simulink model "myrobot"  (R2019b)
settings: Solver=FixedStepAuto  StartTime=0.0  StopTime=2  FixedStep=0.001  MaxStep=0.005  RelTol=1e-3
values from neighbouring files (symbols this model uses):
  g = [0 0 -9.81]    [FK.m]    (also in FK_3DOF.m = [0 0 9.81])
  X = [joint1_pos(1) joint2_pos(1) joint3_pos(1) ee_pos(1)]    [plot_result.m]
  Y = [joint1_pos(2) joint2_pos(2) joint3_pos(2) ee_pos(2)]    [plot_result.m]
  Z = [joint1_pos(3) joint2_pos(3) joint3_pos(3) ee_pos(3)]    [plot_result.m]
libraries: sm_lib x17, nesl_utility x13, robotmaniplib x4, simulink x2
(part 2 of 7)

== matlab function myrobot/DYNAMICS SOLVER/MATLAB Function ==
  data: q input; q_dot input; M output; C output; G output
function [M,C,G] = calculate_dynamics(q,q_dot)

M_func = @(theta1,theta2,theta3)reshape([(sin(theta1).*(-2.272809781200003e-2)+cos(theta1).*sin(theta2).*2.2140098+cos(theta1).*cos(theta2).*sin(theta3).*6.228833385e-1+cos(theta1).*cos(theta3).*sin(theta2).*6.228833385e-1).*(sin(theta1).*(-4.414200000000005e-3)+cos(theta1).*sin(theta2).*(4.3e+1./1.0e+2)+cos(theta1).*cos(theta2).*sin(theta3).*1.20975e-1+cos(theta1).*cos(theta3).*sin(theta2).*1.20975e-1)+sin(theta2).*(cos(theta2).*1.41285e-7+sin(theta2).*2.5374e-1)+cos(theta1).^2.*1.922862803445e-4+sin(theta1).^2.*1.922862803445e-4+(cos(theta2).*cos(theta3)-sin(theta2).*sin(theta3)).*(cos(theta2).*cos(theta3).*1.0425e-2+cos(theta2).*sin(theta3).*2.67415e-8+cos(theta3).*sin(theta2).*2.67415e-8-sin(theta2).*sin(theta3).*1.0425e-2)+(cos(theta1).*2.272809781200003e-2+sin(theta1).*sin(theta2).*2.2140098+cos(theta2).*sin(theta1).*sin(theta3).*6.228833385e-1+cos(theta3).*sin(theta1).*sin(theta2).*6.228833385e-1).*(cos(theta1).*4.414200000000005e-3+sin(theta1).*sin(theta2).*(4.3e+1./1.0e+2)+cos(theta2).*sin(theta1).*sin(theta3).*1.20975e-1+cos(theta3).*sin(theta1).*sin(theta2).*1.20975e-1)+(sin(theta1).*1.4000105183-cos(theta1).*sin(theta2).*1.738546786).*(sin(theta1).*1.719281e-1-cos(theta1).*sin(theta2).*2.13502e-1)+(cos(theta1).*1.4000105183+sin(theta1).*sin(theta2).*1.738546786).*(cos(theta1).*1.719281e-1+sin(theta1).*sin(theta2).*2.13502e-1)+(cos(theta2).*sin(theta3)+cos(theta3).*sin(theta2)).*(cos(theta2).*cos(theta3).*2.67415e-8+cos(theta2).*sin(theta3).*7.5434e-2+cos(theta3).*sin(theta2).*7.5434e-2-sin(theta2).*sin(theta3).*2.67415e-8)+cos(theta2).*(cos(theta2).*2.12824e-2+sin(theta2).*1.41285e-7)+6.04953e-3,-sin(theta1).*((cos(theta2).*cos(theta3)-sin(theta2).*sin(theta3)).*(sin(theta1).*(-2.74946e-3)+cos(theta1).*sin(theta2).*sin(theta3).*2.67415e-8-cos(theta1).*cos(theta2).*cos(theta3).*2.67415e-8+cos(theta1).*cos(theta2).*sin(theta3).*1.0425e-2+cos(theta1).*cos(theta3).*sin(theta2).*1.0425e-2)+(cos(theta2).*sin(theta3)+cos(theta3).*sin(theta2)).*(sin(theta1).*(-2.13561e-9)+cos(theta1).*sin(theta2).*sin(theta3).*7.5434e-2-cos(theta1).*cos(theta2).*cos(theta3).*7.5434e-2+cos(theta1).*cos(theta2).*sin(theta3).*2.67415e-8+cos(theta1).*cos(theta3).*sin(theta2).*2.67415e-8))+cos(theta1).*((cos(theta2).*cos(theta3)-sin(theta2).*sin(theta3)).*(cos(theta1).*2.74946e-3+cos(theta2).*sin(theta1).*sin(theta3).*1.0425e-2+cos(theta3).*sin(theta1).*sin(theta2).*1.0425e-2+sin(theta1).*sin(theta2).*sin(theta3).*2.67415e-8-cos(theta2).*cos(theta3).*sin(theta1).*2.67415e-8)+(cos(theta2).*sin(theta3)+cos(theta3).*sin(theta2)).*(cos(theta1).*2.13561e-9+cos(theta2).*sin(theta1).*sin(theta3).*2.67415e-8+cos(theta3).*sin(theta1).*sin(theta2).*2.67415e-8+sin(theta1).*sin(theta2).*sin(theta3).*7.5434e-2-cos(theta2).*cos(theta3).*sin(theta1).*7.5434e-2))+sin(theta1).*(cos(theta2).*(sin(theta1).*4.99483e-3+cos(theta1).*cos(theta2).*1.41285e-7-cos(theta1).*sin(theta2).*2.12824e-2)-sin(theta2).*(sin(theta1).*7.13886e-8-cos(theta1).*cos(theta2).*2.5374e-1+cos(theta1).*sin(theta2).*1.41285e-7))+cos(theta1).*(cos(theta2).*(cos(theta1).*4.99483e-3-cos(theta2).*sin(theta1).*1.41285e-7+sin(theta1).*sin(theta2).*2.12824e-2)-sin(theta2).*(cos(theta1).*7.13886e-8+cos(theta2).*sin(theta1).*2.5374e-1-sin(theta1).*sin(theta2).*1.41285e-7))-(cos(theta1).*cos(theta2).*2.2140098-cos(theta1).*sin(theta2).*sin(theta3).*6.228833385e-1+cos(theta1).*cos(theta2).*cos(theta3).*6.228833385e-1).*(cos(theta1).*4.414200000000005e-3+sin(theta1).*sin(theta2).*(4.3e+1./1.0e+2)+cos(theta2).*sin(theta1).*sin(theta3).*1.20975e-1+cos(theta3).*sin(theta1).*sin(theta2).*1.20975e-1)+(cos(theta2).*sin(theta1).*2.2140098-sin(theta1).*sin(theta2).*sin(theta3).*6.228833385e-1+cos(theta2).*cos(theta3).*sin(theta1).*6.228833385e-1).*(sin(theta1).*(-4.414200000000005e-3)+cos(theta1).*sin(theta2).*(4.3e+1./1.0e+2)+cos(theta1).*cos(theta2).*sin(theta3).*1.20975e-1+cos(theta1).*cos(theta3).*sin(theta2).*1.20975e-1)-cos(theta1).*cos(theta2).*(cos(theta1).*1.719281e-1+sin(theta1).*sin(theta2).*2.13502e-1).*1.738546786-cos(theta2).*sin(theta1).*(sin(theta1).*1.719281e-1-cos(theta1).*sin(theta2).*2.13502e-1).*1.738546786,(cos(theta1).*sin(theta2).*sin(theta3).*6.228833385e-1-cos(theta1).*cos(theta2).*cos(theta3).*6.228833385e-1).*(cos(theta1).*4.414200000000005e-3+sin(theta1).*sin(theta2).*(4.3e+1./1.0e+2)+cos(theta2).*sin(theta1).*sin(theta3).*1.20975e-1+cos(theta3).*sin(theta1).*sin(theta2).*1.20975e-1)-(sin(theta1).*sin(theta2).*sin(theta3).*6.228833385e-1-cos(theta2).*cos(theta3).*sin(theta1).*6.228833385e-1).*(sin(theta1).*(-4.414200000000005e-3)+cos(theta1).*sin(theta2).*(4.3e+1./1.0e+2)+cos(theta1).*cos(theta2).*sin(theta3).*1.20975e-1+cos(theta1).*cos(theta3).*sin(theta2).*1.20975e-1)-sin(theta1).*((cos(theta2).*cos(theta3)-sin(theta2).*sin(theta3)).*(sin(theta1).*(-2.74946e-3)+cos(theta1).*sin(theta2).*sin(theta3).*2.67415e-8-cos(theta1).*cos(theta2).*cos(theta3).*2.67415e-8+cos(theta1).*cos(theta2).*sin(theta3).*1.0425e-2+cos(theta1).*cos(theta3).*sin(theta2).*1.0425e-2)+(cos(theta2).*sin(theta3)+cos(theta3).*sin(theta2)).*(sin(theta1).*(-2.13561e-9)+cos(theta1).*sin(theta2).*sin(theta3).*7.5434e-2-cos(theta1).*cos(theta2).*cos(theta3).*7.5434e-2+cos(theta1).*cos(theta2).*sin(theta3).*2.67415e-8+cos(theta1).*cos(theta3).*sin(theta2).*2.67415e-8))+cos(theta1).*((cos(theta2).*cos(theta3)-sin(theta2).*sin(theta3)).*(cos(theta1).*2.74946e-3+cos(theta2).*sin(theta1).*sin(theta3).*1.0425e-2+cos(theta3).*sin(theta1).*sin(theta2).*1.0425e-2+sin(theta1).*sin(theta2).*sin(theta3).*2.67415e-8-cos(theta2).*cos(theta3).*sin(theta1).*2.67415e-8)+(cos(theta2).*sin(theta3)+cos(theta3).*sin(theta2)).*(cos(theta1).*2.13561e-9+cos(theta2).*sin(theta1).*sin(theta3).*2.67415e-8+cos(theta3).*sin(theta1).*sin(theta2).*2.67415e-8+sin(theta1).*sin(theta2).*sin(theta3).*7.5434e-2-cos(theta2).*cos(theta3).*sin(theta1).*7.5434e-2)),cos(theta1).*(cos(theta1).*(cos(theta2).*cos(theta3).*2.74946e-3+cos(theta2).*sin(theta3).*2.13561e-9+cos(theta3).*sin(theta2).*2.13561e-9-sin(theta2).*sin(theta3).*2.74946e-3)+(cos(theta2).*sin(theta1).*sin(theta3)+cos(theta3).*sin(theta1).*sin(theta2)).*(cos(theta2).*cos(theta3).*1.0425e-2+cos(theta2).*sin(theta3).*2.67415e-8+cos(theta3).*sin(theta2).*2.67415e-8-sin(theta2).*sin(theta3).*1.0425e-2)+(sin(theta1).*sin(theta2).*sin(theta3)-cos(theta2).*cos(theta3).*sin(theta1)).*(cos(theta2).*cos(theta3).*2.67415e-8+cos(theta2).*sin(theta3).*7.5434e-2+cos(theta3).*sin(theta2).*7.5434e-2-sin(theta2).*sin(theta3).*2.67415e-8))-(cos(theta1).*cos(theta2).*(4.3e+1./1.0e+2)-cos(theta1).*sin(theta2).*sin(theta3).*1.20975e-1+cos(theta1).*cos(theta2).*cos(theta3).*1.20975e-1).*(cos(theta1).*2.272809781200003e-2+sin(theta1).*sin(theta2).*2.2140098+cos(theta2).*sin(theta1).*sin(theta3).*6.228833385e-1+cos(theta3).*sin(theta1).*sin(theta2).*6.228833385e-1)+(cos(theta2).*sin(theta1).*(4.3e+1./1.0e+2)-sin(theta1).*sin(theta2).*sin(theta3).*1.20975e-1+cos(theta2).*cos(theta3).*sin(theta1).*1.20975e-1).*(sin(theta1).*(-2.272809781200003e-2)+cos(theta1).*sin(theta2).*2.2140098+cos(theta1).*cos(theta2).*sin(theta3).*6.228833385e-1+cos(theta1).*cos(theta3).*sin(theta2).*6.228833385e-1)+cos(theta1).*(cos(theta1).*(cos(theta2).*4.99483e-3-sin(theta2).*7.13886e-8)+sin(theta1).*sin(theta2).*(cos(theta2).*2.12824e-2+sin(theta2).*1.41285e-7)-cos(theta2).*sin(theta1).*(cos(theta2).*1.41285e-7+sin(theta2).*2.5374e-1))+sin(theta1).*(sin(theta1).*(cos(theta2).*4.99483e-3-sin(theta2).*7.13886e-8)-cos(theta1).*sin(theta2).*(cos(theta2).*2.12824e-2+sin(theta2).*1.41285e-7)+cos(theta1).*cos(theta2).*(cos(theta2).*1.41285e-7+sin(theta2).*2.5374e-1))-sin(theta1).*(-sin(theta1).*(cos(theta2).*cos(theta3).*2.74946e-3+cos(theta2).*sin(theta3).*2.13561e-9+cos(theta3).*sin(theta2).*2.13561e-9-sin(theta2).*sin(theta3).*2.74946e-3)+(cos(theta1).*sin(theta2).*sin(theta3)-cos(theta1).*cos(theta2).*cos(theta3)).*(cos(theta2).*cos(theta3).*2.67415e-8+cos(theta2).*sin(theta3).*7.5434e-2+cos(theta3).*sin(theta2).*7.5434e-2-sin(theta2).*sin(theta3).*2.67415e-8)+(cos(theta1).*cos(theta2).*sin(theta3)+cos(theta1).*cos(theta3).*sin(theta2)).*(cos(theta2).*cos(theta3).*1.0425e-2+cos(theta2).*sin(theta3).*2.67415e-8+cos(theta3).*sin(theta2).*2.67415e-8-sin(theta2).*sin(theta3).*1.0425e-2))-cos(theta1).*cos(theta2).*(cos(theta1).*1.4000105183+sin(theta1).*sin(theta2).*1.738546786).*2.13502e-1-cos(theta2).*sin(theta1).*(sin(theta1).*1.4000105183-cos(theta1).*sin(theta2).*1.738546786).*2.13502e-1,-sin(theta1).*(sin(theta1).*(sin(theta1).*(sin(theta1).*(-2.47523e-1)+cos(theta1).*cos(theta2).*7.13886e-8+cos(theta1).*sin(theta2).*4.99483e-3)+cos(theta1).*sin(theta2).*(sin(theta1).*4.99483e-3+cos(theta1).*cos(theta2).*1.41285e-7-cos(theta1).*sin(theta2).*2.12824e-2)+cos(theta1).*cos(theta2).*(sin(theta1).*7.13886e-8-cos(theta1).*cos(theta2).*2.5374e-1+cos(theta1).*sin(theta2).*1.41285e-7))+cos(theta1).*(-sin(theta1).*(cos(theta1).*2.47523e-1+cos(theta2).*sin(theta1).*7.13886e-8+sin(theta1).*sin(theta2).*4.99483e-3)+cos(theta1).*sin(theta2).*(cos(theta1).*4.99483e-3-cos(theta2).*sin(theta1).*1.41285e-7+sin(theta1).*sin(theta2).*2.12824e-2)+cos(theta1).*cos(theta2).*(cos(theta1).*7.13886e-8+cos(theta2).*sin(theta1).*2.5374e-1-sin(theta1).*sin(theta2).*1.41285e-7)))+cos(theta1).*(sin(theta1).*(-cos(theta1).*(sin(theta1).*(-2.47523e-1)+cos(theta1).*cos(theta2).*7.13886e-8+cos(theta1).*sin(theta2).*4.99483e-3)+sin(theta1).*sin(theta2).*(sin(theta1).*4.99483e-3+cos(theta1).*cos(theta2).*1.41285e-7-cos(theta1).*sin(theta2).*2.12824e-2)+cos(theta2).*sin(theta1).*(sin(theta1).*7.13886e-8-cos(theta1).*cos(theta2).*2.5374e-1+cos(theta1).*sin(theta2).*1.41285e-7))+cos(theta1).*(cos(theta1).*(cos(theta1).*2.47523e-1+cos(theta2).*sin(theta1).*7.13886e-8+sin(theta1).*sin(theta2).*4.99483e-3)+sin(theta1).*sin(theta2).*(cos(theta1).*4.99483e-3-cos(theta2).*sin(theta1).*1.41285e-7+sin(theta1).*sin(theta2).*2.12824e-2)+cos(theta2).*sin(theta1).*(cos(theta1).*7.13886e-8+cos(theta2).*sin(theta1).*2.5374e-1-sin(theta1).*sin(theta2).*1.41285e-7)))+sin(theta2).^2.*3.71183215904572e-1-cos(theta1).*(sin(theta1).*(cos(theta1).*(sin(theta1).*(-7.44749e-2)+cos(theta1).*sin(theta2).*sin(theta3).*2.13561e-9-cos(theta1).*cos(theta2).*cos(theta3).*2.13561e-9+cos(theta1).*cos(theta2).*sin(theta3).*2.74946e-3+cos(theta1).*cos(theta3).*sin(theta2).*2.74946e-3)+(sin(theta1).*sin(theta2).*sin(theta3)-cos(theta2).*cos(theta3).*sin(theta1)).*(sin(theta1).*(-2.13561e-9)+cos(theta1).*sin(theta2).*sin(theta3).*7.5434e-2-cos(theta1).*cos(theta2).*cos(theta3).*7.5434e-2+cos(theta1).*cos(theta2).*sin(theta3).*2.67415e-8+cos(theta1).*cos(theta3).*sin(theta2).*2.67415e-8)+(cos(theta2).*sin(theta1).*sin(theta3)+cos(theta3).*sin(theta1).*sin(theta2)).*(sin(theta1).*(-2.74946e-3)+cos(theta1).*sin(theta2).*sin(theta3).*2.67415e-8-cos(theta1).*cos(theta2).*cos(theta3).*2.67415e-8+cos(theta1).*cos(theta2).*sin(theta3).*1.0425e-2+cos(theta1).*cos(theta3).*sin(theta2).*1.0425e-2))-cos(theta1).*((cos(theta2).*sin(theta1).*sin(theta3)+cos(theta3).*sin(theta1).*sin(theta2)).*(cos(theta1).*2.74946e-3+cos(theta2).*sin(theta1).*sin(theta3).*1.0425e-2+cos(theta3).*sin(theta1).*sin(theta2).*1.0425e-2+sin(theta1).*sin(theta2).*sin(theta3).*2.67415e-8-cos(theta2).*cos(theta3).*sin(theta1).*2.67415e-8)+cos(theta1).*(cos(theta1).*7.44749e-2+cos(theta2).*sin(theta1).*sin(theta3).*2.74946e-3+cos(theta3).*sin(theta1).*sin(theta2).*2.74946e-3+sin(theta1).*sin(theta2).*sin(theta3).*2.13561e-9-cos(theta2).*cos(theta3).*sin(theta1).*2.13561e-9)+(sin(theta1).*sin(theta2).*sin(theta3)-cos(theta2).*cos(theta3).*sin(theta1)).*(cos(theta1).*2.13561e-9+cos(theta2).*sin(theta1).*sin(theta3).*2.67415e-8+cos(theta3).*sin(theta1).*sin(theta2).*2.67415e-8+sin(theta1).*sin(theta2).*sin(theta3).*7.5434e-2-cos(theta2).*cos(theta3).*sin(theta1).*7.5434e-2)))+(cos(theta1).*cos(theta2).*(4.3e+1./1.0e+2)-cos(theta1).*sin(theta2).*sin(theta3).*1.20975e-1+cos(theta1).*cos(theta2).*cos(theta3).*1.20975e-1).*(cos(theta1).*cos(theta2).*2.2140098-cos(theta1).*sin(theta2).*sin(theta3).*6.228833385e-1+cos(theta1).*cos(theta2).*cos(theta3).*6.228833385e-1)+(sin(theta2).*2.2140098+cos(theta2).*sin(theta3).*6.228833385e-1+cos(theta3).*sin(theta2).*6.228833385e-1).*(sin(theta2).*(4.3e+1./1.0e+2)+cos(theta2).*sin(theta3).*1.20975e-1+cos(theta3).*sin(theta2).*1.20975e-1)+cos(theta1).^2.*cos(theta2).^2.*3.71183215904572e-1+cos(theta2).^2.*sin(theta1).^2.*3.71183215904572e-1-sin(theta1).*(cos(theta1).*(-sin(theta1).*(cos(theta1).*7.44749e-2+cos(theta2).*sin(theta1).*sin(theta3).*2.74946e-3+cos(theta3).*sin(theta1).*sin(theta2).*2.74946e-3+sin(theta1).*sin(theta2).*sin(theta3).*2.13561e-9-cos(theta2).*cos(theta3).*sin(theta1).*2.13561e-9)+(cos(theta1).*sin(theta2).*sin(theta3)-cos(theta1).*cos(theta2).*cos(theta3)).*(cos(theta1).*2.13561e-9+cos(theta2).*sin(theta1).*sin(theta3).*2.67415e-8+cos(theta3).*sin(theta1).*sin(theta2).*2.67415e-8+sin(theta1).*sin(theta2).*sin(theta3).*7.5434e-2-cos(theta2).*cos(theta3).*sin(theta1).*7.5434e-2)+(cos(theta1).*cos(theta2).*sin(theta3)+cos(theta1).*cos(theta3).*sin(theta2)).*(cos(theta1).*2.74946e-3+cos(theta2).*sin(theta1).*sin(theta3).*1.0425e-2+cos(theta3).*sin(theta1).*sin(theta2).*1.0425e-2+sin(theta1).*sin(theta2).*sin(theta3).*2.67415e-8-cos(theta2).*cos(theta3).*sin(theta1).*2.67415e-8))-sin(theta1).*(-sin(theta1).*(sin(theta1).*(-7.44749e-2)+cos(theta1).*sin(theta2).*sin(theta3).*2.13561e-9-cos(theta1).*cos(theta2).*cos(theta3).*2.13561e-9+cos(theta1).*cos(theta2).*sin(theta3).*2.74946e-3+cos(theta1).*cos(theta3).*sin(theta2).*2.74946e-3)+(cos(theta1).*sin(theta2).*sin(theta3)-cos(theta1).*cos(theta2).*cos(theta3)).*(sin(theta1).*(-2.13561e-9)+cos(theta1).*sin(theta2).*sin(theta3).*7.5434e-2-cos(theta1).*cos(theta2).*cos(theta3).*7.5434e-2+cos(theta1).*cos(theta2).*sin(theta3).*2.67415e-8+cos(theta1).*cos(theta3).*sin(theta2).*2.67415e-8)+(cos(theta1).*cos(theta2).*sin(theta3)+cos(theta1).*cos(theta3).*sin(theta2)).*(sin(theta1).*(-2.74946e-3)+cos(theta1).*sin(theta2).*sin(theta3).*2.67415e-8-cos(theta1).*cos(theta2).*cos(theta3).*2.67415e-8+cos(theta1).*cos(theta2).*sin(theta3).*1.0425e-2+cos(theta1).*cos(theta3).*sin(theta2).*1.0425e-2)))+(cos(theta2).*sin(theta1).*2.2140098-sin(theta1).*sin(theta2).*sin(theta3).*6.228833385e-1+cos(theta2).*cos(theta3).*sin(theta1).*6.228833385e-1).*(cos(theta2).*sin(theta1).*(4.3e+1./1.0e+2)-sin(theta1).*sin(theta2).*sin(theta3).*1.20975e-1+cos(theta2).*cos(theta3).*sin(theta1).*1.20975e-1),-(cos(theta1).*sin(theta2).*sin(theta3).*6.228833385e-1-cos(theta1).*cos(theta2).*cos(theta3).*6.228833385e-1).*(cos(theta1).*cos(theta2).*(4.3e+1./1.0e+2)-cos(theta1).*sin(theta2).*sin(theta3).*1.20975e-1+cos(theta1).*cos(theta2).*cos(theta3).*1.20975e-1)-cos(theta1).*(sin(theta1).*(cos(theta1).*(sin(theta1).*(-7.44749e-2)+cos(theta1).*sin(theta2).*sin(theta3).*2.13561e-9-cos(theta1).*cos(theta2).*cos(theta3).*2.13561e-9+cos(theta1).*cos(theta2).*sin(theta3).*2.74946e-3+cos(theta1).*cos(theta3).*sin(theta2).*2.74946e-3)+(sin(theta1).*sin(theta2).*sin(theta3)-cos(theta2).*cos(theta3).*sin(theta1)).*(sin(theta1).*(-2.13561e-9)+cos(theta1).*sin(theta2).*sin(theta3).*7.5434e-2-cos(theta1).*cos(theta2).*cos(theta3).*7.5434e-2+cos(theta1).*cos(theta2).*sin(theta3).*2.67415e-8+cos(theta1).*cos(theta3).*sin(theta2).*2.67415e-8)+(cos(theta2).*sin(theta1).*sin(theta3)+cos(theta3).*sin(theta1).*sin(theta2)).*(sin(theta1).*(-2.74946e-3)+cos(theta1).*sin(theta2).*sin(theta3).*2.67415e-8-cos(theta1).*cos(theta2).*cos(theta3).*2.67415e-8+cos(theta1).*cos(theta2).*sin(theta3).*1.0425e-2+cos(theta1).*cos(theta3).*sin(theta2).*1.0425e-2))-cos(theta1).*((cos(theta2).*sin(theta1).*sin(theta3)+cos(theta3).*sin(theta1).*sin(theta2)).*(cos(theta1).*2.74946e-3+cos(theta2).*sin(theta1).*sin(theta3).*1.0425e-2+cos(theta3).*sin(theta1).*sin(theta2).*1.0425e-2+sin(theta1).*sin(theta2).*sin(theta3).*2.67415e-8-cos(theta2).*cos(theta3).*sin(theta1).*2.67415e-8)+cos(theta1).*(cos(theta1).*7.44749e-2+cos(theta2).*sin(theta1).*sin(theta3).*2.74946e-3+cos(theta3).*sin(theta1).*sin(theta2).*2.74946e-3+sin(theta1).*sin(theta2).*sin(theta3).*2.13561e-9-cos(theta2).*cos(theta3).*sin(theta1).*2.13561e-9)+(sin(theta1).*sin(theta2).*sin(theta3)-cos(theta2).*cos(theta3).*sin(theta1)).*(cos(theta1).*2.13561e-9+cos(theta2).*sin(theta1).*sin(theta3).*2.67415e-8+cos(theta3).*sin(theta1).*sin(theta2).*2.67415e-8+sin(theta1).*sin(theta2).*sin(theta3).*7.5434e-2-cos(theta2).*cos(theta3).*sin(theta1).*7.5434e-2)))-(sin(theta1).*sin(theta2).*sin(theta3).*6.228833385e-1-cos(theta2).*cos(theta3).*sin(theta1).*6.228833385e-1).*(cos(theta2).*sin(theta1).*(4.3e+1./1.0e+2)-sin(theta1).*sin(theta2).*sin(theta3).*1.20975e-1+cos(theta2).*cos(theta3).*sin(theta1).*1.20975e-1)+(cos(theta2).*sin(theta3).*6.228833385e-1+cos(theta3).*sin(theta2).*6.228833385e-1).*(sin(theta2).*(4.3e+1./1.0e+2)+cos(theta2).*sin(theta3).*1.20975e-1+cos(theta3).*sin(theta2).*1.20975e-1)-sin(theta1).*(cos(theta1).*(-sin(theta1).*(cos(theta1).*7.44749e-2+cos(theta2).*sin(theta1).*sin(theta3).*2.74946e-3+cos(theta3).*sin(theta1).*sin(theta2).*2.74946e-3+sin(theta1).*sin(theta2).*sin(theta3).*2.13561e-9-cos(theta2).*cos(theta3).*sin(theta1).*2.13561e-9)+(cos(theta1).*sin(theta2).*sin(theta3)-cos(theta1).*cos(theta2).*cos(theta3)).*(cos(theta1).*2.13561e-9+cos(theta2).*sin(theta1).*sin(theta3).*2.67415e-8+cos(theta3).*sin(theta1).*sin(theta2).*2.67415e-8+sin(theta1).*sin(theta2).*sin(theta3).*7.5434e-2-cos(theta2).*cos(theta3).*sin(theta1).*7.5434e-2)+(cos(theta1).*cos(theta2).*sin(theta3)+cos(theta1).*cos(theta3).*sin(theta2)).*(cos(theta1).*2.74946e-3+cos(theta2).*sin(theta1).*sin(theta3).*1.0425e-2+cos(theta3).*sin(theta1).*sin(theta2).*1.0425e-2+sin(theta1).*sin(theta2).*sin(theta3).*2.67415e-8-cos(theta2).*cos(theta3).*sin(theta1).*2.67415e-8))-sin(theta1).*(-sin(theta1).*(sin(theta1).*(-7.44749e-2)+cos(theta1).*sin(theta2).*sin(theta3).*2.13561e-9-cos(theta1).*cos(theta2).*cos(theta3).*2.13561e-9+cos(theta1).*cos(theta2).*sin(theta3).*2.74946e-3+cos(theta1).*cos(theta3).*sin(theta2).*2.74946e-3)+(cos(theta1).*sin(theta2).*sin(theta3)-cos(theta1).*cos(theta2).*cos(theta3)).*(sin(theta1).*(-2.13561e-9)+cos(theta1).*sin(theta2).*sin(theta3).*7.5434e-2-cos(theta1).*cos(theta2).*cos(theta3).*7.5434e-2+cos(theta1).*cos(theta2).*sin(theta3).*2.67415e-8+cos(theta1).*cos(theta3).*sin(theta2).*2.67415e-8)+(cos(theta1).*cos(theta2).*sin(theta3)+cos(theta1).*cos(theta3).*sin(theta2)).*(sin(theta1).*(-2.74946e-3)+cos(theta1).*sin(theta2).*sin(theta3).*2.67415e-8-cos(theta1).*cos(theta2).*cos(theta3).*2.67415e-8+cos(theta1).*cos(theta2).*sin(theta3).*1.0425e-2+cos(theta1).*cos(theta3).*sin(theta2).*1.0425e-2))),cos(theta1).*(cos(theta1).*(cos(theta2).*cos(theta3).*2.74946e-3+cos(theta2).*sin(theta3).*2.13561e-9+cos(theta3).*sin(theta2).*2.13561e-9-sin(theta2).*sin(theta3).*2.74946e-3)+(cos(theta2).*sin(theta1).*sin(theta3)+cos(theta3).*sin(theta1).*sin(theta2)).*(cos(theta2).*cos(theta3).*1.0425e-2+cos(theta2).*sin(theta3).*2.67415e-8+cos(theta3).*sin(theta2).*2.67415e-8-sin(theta2).*sin(theta3).*1.0425e-2)+(sin(theta1).*sin(theta2).*sin(theta3)-cos(theta2).*cos(theta3).*sin(theta1)).*(cos(theta2).*cos(theta3).*2.67415e-8+cos(theta2).*sin(theta3).*7.5434e-2+cos(theta3).*sin(theta2).*7.5434e-2-sin(theta2).*sin(theta3).*2.67415e-8))+(cos(theta1).*sin(theta2).*sin(theta3).*1.20975e-1-cos(theta1).*cos(theta2).*cos(theta3).*1.20975e-1).*(cos(theta1).*2.272809781200003e-2+sin(theta1).*sin(theta2).*2.2140098+cos(theta2).*sin(theta1).*sin(theta3).*6.228833385e-1+cos(theta3).*sin(theta1).*sin(theta2).*6.228833385e-1)-(sin(theta1).*sin(theta2).*sin(theta3).*1.20975e-1-cos(theta2).*cos(theta3).*sin(theta1).*1.20975e-1).*(sin(theta1).*(-2.272809781200003e-2)+cos(theta1).*sin(theta2).*2.2140098+cos(theta1).*cos(theta2).*sin(theta3).*6.228833385e-1+cos(theta1).*cos(theta3).*sin(theta2).*6.228833385e-1)-sin(theta1).*(-sin(theta1).*(cos(theta2).*cos(theta3).*2.74946e-3+cos(theta2).*sin(theta3).*2.13561e-9+cos(theta3).*sin(theta2).*2.13561e-9-sin(theta2).*sin(theta3).*2.74946e-3)+(cos(theta1).*sin(theta2).*sin(theta3)-cos(theta1).*cos(theta2).*cos(theta3)).*(cos(theta2).*cos(theta3).*2.67415e-8+cos(theta2).*sin(theta3).*7.5434e-2+cos(theta3).*sin(theta2).*7.5434e-2-sin(theta2).*sin(theta3).*2.67415e-8)+(cos(theta1).*cos(theta2).*sin(theta3)+cos(theta1).*cos(theta3).*sin(theta2)).*(cos(theta2).*cos(theta3).*1.0425e-2+cos(theta2).*sin(theta3).*2.67415e-8+cos(theta3).*sin(theta2).*2.67415e-8-sin(theta2).*sin(theta3).*1.0425e-2)),-cos(theta1).*(sin(theta1).*(cos(theta1).*(sin(theta1).*(-7.44749e-2)+cos(theta1).*sin(theta2).*sin(theta3).*2.13561e-9-cos(theta1).*cos(theta2).*cos(theta3).*2.13561e-9+cos(theta1).*cos(theta2).*sin(theta3).*2.74946e-3+cos(theta1).*cos(theta3).*sin(theta2).*2.74946e-3)+(sin(theta1).*sin(theta2).*sin(theta3)-cos(theta2).*cos(theta3).*sin(theta1)).*(sin(theta1).*(-2.13561e-9)+cos(theta1).*sin(theta2).*sin(theta3).*7.5434e-2-cos(theta1).*cos(theta2).*cos(theta3).*7.5434e-2+cos(theta1).*cos(theta2).*sin(theta3).*2.67415e-8+cos(theta1).*cos(theta3).*sin(theta2).*2.67415e-8)+(cos(theta2).*sin(theta1).*sin(theta3)+cos(theta3).*sin(theta1).*sin(theta2)).*(sin(theta1).*(-2.74946e-3)+cos(theta1).*sin(theta2).*sin(theta3).*2.67415e-8-cos(theta1).*cos(theta2).*cos(theta3).*2.67415e-8+cos(theta1).*cos(theta2).*sin(theta3).*1.0425e-2+cos(theta1).*cos(theta3).*sin(theta2).*1.0425e-2))-cos(theta1).*((cos(theta2).*sin(theta1).*sin(theta3)+cos(theta3).*sin(theta1).*sin(theta2)).*(cos(theta1).*2.74946e-3+cos(theta2).*sin(theta1).*sin(theta3).*1.0425e-2+cos(theta3).*sin(theta1).*sin(theta2).*1.0425e-2+sin(theta1).*sin(theta2).*sin(theta3).*2.67415e-8-cos(theta2).*cos(theta3).*sin(theta1).*2.67415e-8)+cos(theta1).*(cos(theta1).*7.44749e-2+cos(theta2).*sin(theta1).*sin(theta3).*2.74946e-3+cos(theta3).*sin(theta1).*sin(theta2).*2.74946e-3+sin(theta1).*sin(theta2).*sin(theta3).*2.13561e-9-cos(theta2).*cos(theta3).*sin(theta1).*2.13561e-9)+(sin(theta1).*sin(theta2).*sin(theta3)-cos(theta2).*cos(theta3).*sin(theta1)).*(cos(theta1).*2.13561e-9+cos(theta2).*sin(theta1).*sin(theta3).*2.67415e-8+cos(theta3).*sin(theta1).*sin(theta2).*2.67415e-8+sin(theta1).*sin(theta2).*sin(theta3).*7.5434e-2-cos(theta2).*cos(theta3).*sin(theta1).*7.5434e-2)))+(cos(theta2).*sin(theta3).*1.20975e-1+cos(theta3).*sin(theta2).*1.20975e-1).*(sin(theta2).*2.2140098+cos(theta2).*sin(theta3).*6.228833385e-1+cos(theta3).*sin(theta2).*6.228833385e-1)-(cos(theta1).*sin(theta2).*sin(theta3).*1.20975e-1-cos(theta1).*cos(theta2).*cos(theta3).*1.20975e-1).*(cos(theta1).*cos(theta2).*2.2140098-cos(theta1).*sin(theta2).*sin(theta3).*6.228833385e-1+cos(theta1).*cos(theta2).*cos(theta3).*6.228833385e-1)-(sin(theta1).*sin(theta2).*sin(theta3).*1.20975e-1-cos(theta2).*cos(theta3).*sin(theta1).*1.20975e-1).*(cos(theta2).*sin(theta1).*2.2140098-sin(theta1).*sin(theta2).*sin(theta3).*6.228833385e-1+cos(theta2).*cos(theta3).*sin(theta1).*6.228833385e-1)-sin(theta1).*(cos(theta1).*(-sin(theta1).*(cos(theta1).*7.44749e-2+cos(theta2).*sin(theta1).*sin(theta3).*2.74946e-3+cos(theta3).*sin(theta1).*sin(theta2).*2.74946e-3+sin(theta1).*sin(theta2).*sin(theta3).*2.13561e-9-cos(theta2).*cos(theta3).*sin(theta1).*2.13561e-9)+(cos(theta1).*sin(theta2).*sin(theta3)-cos(theta1).*cos(theta2).*cos(theta3)).*(cos(theta1).*2.13561e-9+cos(theta2).*sin(theta1).*sin(theta3).*2.67415e-8+cos(theta3).*sin(theta1).*sin(theta2).*2.67415e-8+sin(theta1).*sin(theta2).*sin(theta3).*7.5434e-2-cos(theta2).*cos(theta3).*sin(theta1).*7.5434e-2)+(cos(theta1).*cos(theta2).*sin(theta3)+cos(theta1).*cos(theta3).*sin(theta2)).*(cos(theta1).*2.74946e-3+cos(theta2).*sin(theta1).*sin(theta3).*1.0425e-2+cos(theta3).*sin(theta1).*sin(theta2).*1.0425e-2+sin(theta1).*sin(theta2).*sin(theta3).*2.67415e-8-cos(theta2).*cos(theta3).*sin(theta1).*2.67415e-8))-sin(theta1).*(-sin(theta1).*(sin(theta1).*(-7.44749e-2)+cos(theta1).*sin(theta2).*sin(theta3).*2.13561e-9-cos(theta1).*cos(theta2).*cos(theta3).*2.13561e-9+cos(theta1).*cos(theta2).*sin(theta3).*2.74946e-3+cos(theta1).*cos(theta3).*sin(theta2).*2.74946e-3)+(cos(theta1).*sin(theta2).*sin(theta3)-cos(theta1).*cos(theta2).*cos(theta3)).*(sin(theta1).*(-2.13561e-9)+cos(theta1).*sin(theta2).*sin(theta3).*7.5434e-2-cos(theta1).*cos(theta2).*cos(theta3).*7.5434e-2+cos(theta1).*cos(theta2).*sin(theta3).*2.67415e-8+cos(theta1).*cos(theta3).*sin(theta2).*2.67415e-8)+(cos(theta1).*cos(theta2).*sin(theta3)+cos(theta1).*cos(theta3).*sin(theta2)).*(sin(theta1).*(-2.74946e-3)+cos(theta1).*sin(theta2).*sin(theta3).*2.67415e-8-cos(theta1).*cos(theta2).*cos(theta3).*2.67415e-8+cos(theta1).*cos(theta2).*sin(theta3).*1.0425e-2+cos(theta1).*cos(theta3).*sin(theta2).*1.0425e-2))),(sin(theta1).*sin(theta2).*sin(theta3).*1.20975e-1-cos(theta2).*cos(theta3).*sin(theta1).*1.20975e-1).*(sin(theta1).*sin(theta2).*sin(theta3).*6.228833385e-1-cos(theta2).*cos(theta3).*sin(theta1).*6.228833385e-1)-cos(theta1).*(sin(theta1).*(cos(theta1).*(sin(theta1).*(-7.44749e-2)+cos(theta1).*sin(theta2).*sin(theta3).*2.13561e-9-cos(theta1).*cos(theta2).*cos(theta3).*2.13561e-9+cos(theta1).*cos(theta2).*sin(theta3).*2.74946e-3+cos(theta1).*cos(theta3).*sin(theta2).*2.74946e-3)+(sin(theta1).*sin(theta2).*sin(theta3)-cos(theta2).*cos(theta3).*sin(theta1)).*(sin(theta1).*(-2.13561e-9)+cos(theta1).*sin(theta2).*sin(theta3).*7.5434e-2-cos(theta1).*cos(theta2).*cos(theta3).*7.5434e-2+cos(theta1).*cos(theta2).*sin(theta3).*2.67415e-8+cos(theta1).*cos(theta3).*sin(theta2).*2.67415e-8)+(cos(theta2).*sin(theta1).*sin(theta3)+cos(theta3).*sin(theta1).*sin(theta2)).*(sin(theta1).*(-2.74946e-3)+cos(theta1).*sin(theta2).*sin(theta3).*2.67415e-8-cos(theta1).*cos(theta2).*cos(theta3).*2.67415e-8+cos(theta1).*cos(theta2).*sin(theta3).*1.0425e-2+cos(theta1).*cos(theta3).*sin(theta2).*1.0425e-2))-cos(theta1).*((cos(theta2).*sin(theta1).*sin(theta3)+cos(theta3).*sin(theta1).*sin(theta2)).*(cos(theta1).*2.74946e-3+cos(theta2).*sin(theta1).*sin(theta3).*1.0425e-2+cos(theta3).*sin(theta1).*sin(theta2).*1.0425e-2+sin(theta1).*sin(theta2).*sin(theta3).*2.67415e-8-cos(theta2).*cos(theta3).*sin(theta1).*2.67415e-8)+cos(theta1).*(cos(theta1).*7.44749e-2+cos(theta2).*sin(theta1).*sin(theta3).*2.74946e-3+cos(theta3).*sin(theta1).*sin(theta2).*2.74946e-3+sin(theta1).*sin(theta2).*sin(theta3).*2.13561e-9-cos(theta2).*cos(theta3).*sin(theta1).*2.13561e-9)+(sin(theta1).*sin(theta2).*sin(theta3)-cos(theta2).*cos(theta3).*sin(theta1)).*(cos(theta1).*2.13561e-9+cos(theta2).*sin(theta1).*sin(theta3).*2.67415e-8+cos(theta3).*sin(theta1).*sin(theta2).*2.67415e-8+sin(theta1).*sin(theta2).*sin(theta3).*7.5434e-2-cos(theta2).*cos(theta3).*sin(theta1).*7.5434e-2)))+(cos(theta2).*sin(theta3).*1.20975e-1+cos(theta3).*sin(theta2).*1.20975e-1).*(cos(theta2).*sin(theta3).*6.228833385e-1+cos(theta3).*sin(theta2).*6.228833385e-1)-sin(theta1).*(cos(theta1).*(-sin(theta1).*(cos(theta1).*7.44749e-2+cos(theta2).*sin(theta1).*sin(theta3).*2.74946e-3+cos(theta3).*sin(theta1).*sin(theta2).*2.74946e-3+sin(theta1).*sin(theta2).*sin(theta3).*2.13561e-9-cos(theta2).*cos(theta3).*sin(theta1).*2.13561e-9)+(cos(theta1).*sin(theta2).*sin(theta3)-cos(theta1).*cos(theta2).*cos(theta3)).*(cos(theta1).*2.13561e-9+cos(theta2).*sin(theta1).*sin(theta3).*2.67415e-8+cos(theta3).*sin(theta1).*sin(theta2).*2.67415e-8+sin(theta1).*sin(theta2).*sin(theta3).*7.5434e-2-cos(theta2).*cos(theta3).*sin(theta1).*7.5434e-2)+(cos(theta1).*cos(theta2).*sin(theta3)+cos(theta1).*cos(theta3).*sin(theta2)).*(cos(theta1).*2.74946e-3+cos(theta2).*sin(theta1).*sin(theta3).*1.0425e-2+cos(theta3).*sin(theta1).*sin(theta2).*1.0425e-2+sin(theta1).*sin(theta2).*sin(theta3).*2.67415e-8-cos(theta2).*cos(theta3).*sin(theta1).*2.67415e-8))-sin(theta1).*(-sin(theta1).*(sin(theta1).*(-7.44749e-2)+cos(theta1).*sin(theta2).*sin(theta3).*2.13561e-9-cos(theta1).*cos(theta2).*cos(theta3).*2.13561e-9+cos(theta1).*cos(theta2).*sin(theta3).*2.74946e-3+cos(theta1).*cos(theta3).*sin(theta2).*2.74946e-3)+(cos(theta1).*sin(theta2).*sin(theta3)-cos(theta1).*cos(theta2).*cos(theta3)).*(sin(theta1).*(-2.13561e-9)+cos(theta1).*sin(theta2).*sin(theta3).*7.5434e-2-cos(theta1).*cos(theta2).*cos(theta3).*7.5434e-2+cos(theta1).*cos(theta2).*sin(theta3).*2.67415e-8+cos(theta1).*cos(theta3).*sin(theta2).*2.67415e-8)+(cos(theta1).*cos(theta2).*sin(theta3)+cos(theta1).*cos(theta3).*sin(theta2)).*(sin(theta1).*(-2.74946e-3)+cos(theta1).*sin(theta2).*sin(theta3).*2.67415e-8-cos(theta1).*cos(theta2).*cos(theta3).*2.67415e-8+cos(theta1).*cos(theta2).*sin(theta3).*1.0425e-2+cos(theta1).*cos(theta3).*sin(theta2).*1.0425e-2)))+(cos(theta1).*sin(theta2).*sin(theta3).*1.20975e-1-cos(theta1).*cos(theta2).*cos(theta3).*1.20975e-1).*(cos(theta1).*sin(theta2).*sin(theta3).*6.228833385e-1-cos(theta1).*cos(theta2).*cos(theta3).*6.228833385e-1)],[3,3]);
